simulink model "FBL_UAV_Final_All"  (R2024b)
settings: Solver=ode45  StartTime=0.0  StopTime=3  MaxStep=0.001  RelTol=1e-3
undefined symbols (not defined in the file): A, A_inv, B, Q, R
libraries: slpidlib x8, mpclib x1, rllib x1, simulink x1
(part 1 of 2)
settings Model: Creator=shree  LastModifiedBy=shree
settings SolverCC: MaxConsecutiveMinStep=5
settings RTWCC: GenerateReport=on  LaunchReport=on

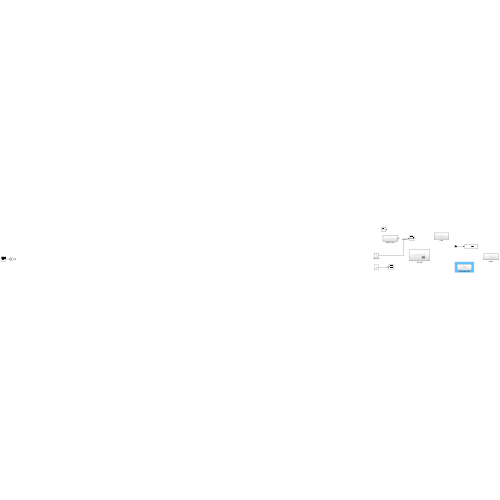
[thumbnail: Simulink's stored preview of the top-level diagram]
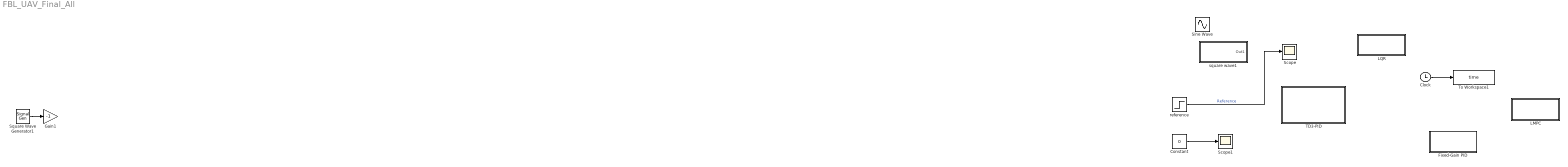
== system FBL_UAV_Final_All ==
  Clock : Clock
      settings: Decimation=4
  Constant : Constant  Value=0
  Fixed-Gain PID : Subsystem
  Gain1 : Gain  Gain=-1
  LMPC : Subsystem
  LQR : Subsystem
  Scope : Scope
  Scope1 : Scope
  Sine Wave : Sin  Amplitude=3  Frequency=3  SampleTime=0
  Square Wave Generator1 : SignalGenerator  WaveForm=square  Amplitude=3
  TD3-PID : Subsystem
  To Workspace1 : ToWorkspace  VariableName=time  SaveFormat=Timeseries  SampleTime=-1
  reference : Step  Time=0.5  SampleTime=0.1
  square wave1 : Subsystem
  wires:
  Square Wave Generator1/1 -> Gain1/1
  Clock/1 -> To Workspace1/1
  Constant/1 -> Scope1/1
  reference/1 -> Scope/1  "Reference"

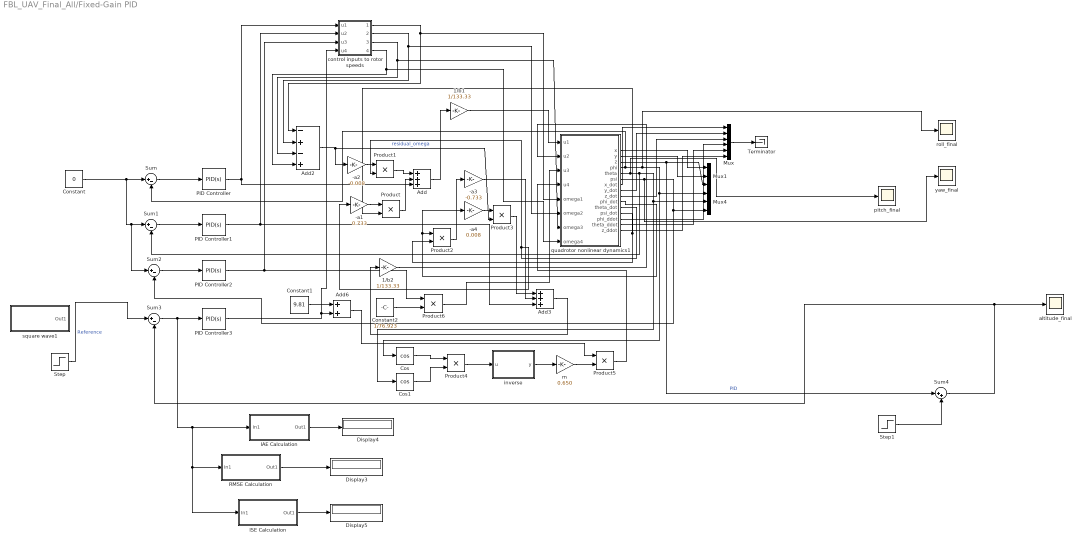
== system FBL_UAV_Final_All/Fixed-Gain PID ==
  -a1 : Gain  Gain=0.733
  -a2 : Gain  Gain=-0.008
  -a3 : Gain  Gain=-0.733
  -a4 : Gain  Gain=0.008
  1/b1 : Gain  Gain=1/133.33
  1/b2 : Gain  Gain=1/133.33
  Add : Sum  Inputs=+++
  Add2 : Sum  Inputs=-+-+
  Add3 : Sum  Inputs=+++
  Add6 : Sum
  Constant : Constant  Value=0
  Constant1 : Constant  Value=9.81
  Constant2 : Constant  Value=1/76.923
  Cos : Trigonometry  Operator=cos
  Cos1 : Trigonometry  Operator=cos
  Display3 : Display
  Display4 : Display
  Display5 : Display
  IAE Calculation : Subsystem
  ISE Calculation : Subsystem
  Mux : Mux  Inputs=6
  Mux1 : Mux  Inputs=3
  Mux4 : Mux  Inputs=3
  PID Controller : slpidlib/PID Controller  Controller=PID  Form=Parallel  TimeDomain=Continuous-time  UseExternalTs=off  SampleTime=-1  IntegratorMethod=Forward Euler  FilterMethod=Forward Euler  ControllerParametersSource=internal  P=50  I=50  UseKiTs=off  D=50  UseExternalDerivativeSource=off  N=200  UseFilter=on  TunerSelectOption=Transfer Function Based (PID Tuner App)  InitialConditionSource=internal  InitialConditionForIntegrator=0  InitialConditionForFilter=0  DifferentiatorICPrevScaledInput=0  ExternalReset=none  TrackingMode=off  Kt=1  LimitOutput=off  SatLimitsSource=internal  UpperSaturationLimit=inf  LowerSaturationLimit=-inf  LinearizeAsGain=on  AntiWindupMode=none  Kb=1  LimitIntegrator=off  UpperIntegratorSaturationLimit=inf  LowerIntegratorSaturationLimit=-inf  POutMin=[]  POutMax=[]  IOutMin=[]  IOutMax=[]  DOutMin=[]  DOutMax=[]  NOutMin=[]  NOutMax=[]  SumOutMin=[]  SumOutMax=[]  SaturationOutMin=[]  SaturationOutMax=[]  PParamMin=[]  PParamMax=[]  IParamMin=[]  IParamMax=[]  DParamMin=[]  DParamMax=[]  NParamMin=[]  NParamMax=[]  KbParamMin=[]  KbParamMax=[]  KtParamMin=[]  KtParamMax=[]  KbOutMin=[]  KbOutMax=[]  KtOutMin=[]  KtOutMax=[]  IntegratorOutMin=[]  IntegratorOutMax=[]  FilterOutMin=[]  FilterOutMax=[]  SumI1OutMin=[]  SumI1OutMax=[]  SumI2OutMin=[]  SumI2OutMax=[]  SumI3OutMin=[]  SumI3OutMax=[]  SumI4OutMin=[]  SumI4OutMax=[]  SumDOutMin=[]  SumDOutMax=[]  DifferentiatorOutMin=[]  DifferentiatorOutMax=[]  FilterDiffOutCoefMin=[]  FilterDiffOutCoefMax=[]  ReciprocalOutMin=[]  ReciprocalOutMax=[]  SumDenOutMin=[]  SumDenOutMax=[]  SumNumOutMin=[]  SumNumOutMax=[]  DivideOutMin=[]  DivideOutMax=[]  UdiffTsProdOutMin=[]  UdiffTsProdOutMax=[]  NTsProdOutMin=[]  NTsProdOutMax=[]  UintegralTsProdOutMin=[]  UintegralTsProdOutMax=[]  UngainTsProdOutMin=[]  UngainTsProdOutMax=[]  ClampingZeroOutDataTypeStr=Inherit: Inherit via back propagation  ClampingZeroOutMin=[]  ClampingZeroOutMax=[]  FilterDenConstantOutDataTypeStr=Inherit: Inherit via back propagation  FilterDenConstantOutMin=[]  FilterDenConstantOutMax=[]  PCopyOutDataTypeStr=Inherit: Inherit via back propagation  PCopyOutMin=[]  PCopyOutMax=[]  NCopyOutDataTypeStr=Inherit: Inherit via back propagation  NCopyOutMin=[]  NCopyOutMax=[]  IntegratorContinuousStateAttributes=''  IntegratorStateMustResolveToSignalObject=off  IntegratorRTWStateStorageClass=Auto  FilterContinuousStateAttributes=''  FilterStateMustResolveToSignalObject=off  FilterRTWStateStorageClass=Auto  ParallelPVariant=InternalParameters  IdealPVariant=Disabled  IVariant=InternalParameters  DVariant=InternalParameters  IntegratorVariant=Continuous  SatVariant=Disabled  AWVariant=Passthrough  PCopyVariant=Disabled  TRVariant=Disabled  FdbkBlocksVariant=Forward  IdealPFdbkVariant=Disabled  SatFdbkVariant=Disabled  DerivativeFilterVariant=ContFilter  NVariant=InternalParameters  NCopyVariant=Disabled  FilterICVariant=InternalICsFilter  IntegratorICVariant=InternalICs  ExternalResetVariant=Disabled  TRSumVariant=Passthrough  SumFdbkVariant=Disabled  SumVariant=Sum_PID  TsampFilterVariant=InternalTs  TsampNgainVariant=Passthrough  TsampIntegralVariant=Disabled_SignalSpec  ExternalSaturationOutDataTypeStr=Inherit: Same as second input  DerivativeSourceVariant=ErrorSignal  PreIntVariant=InternalPreInt
  PID Controller1 : slpidlib/PID Controller  Controller=PID  Form=Parallel  TimeDomain=Continuous-time  UseExternalTs=off  SampleTime=-1  IntegratorMethod=Forward Euler  FilterMethod=Forward Euler  ControllerParametersSource=internal  P=10  I=0.5  UseKiTs=off  D=10  UseExternalDerivativeSource=off  N=100  UseFilter=on  TunerSelectOption=Transfer Function Based (PID Tuner App)  InitialConditionSource=internal  InitialConditionForIntegrator=0  InitialConditionForFilter=0  DifferentiatorICPrevScaledInput=0  ExternalReset=none  TrackingMode=off  Kt=1  LimitOutput=off  SatLimitsSource=internal  UpperSaturationLimit=inf  LowerSaturationLimit=-inf  LinearizeAsGain=on  AntiWindupMode=none  Kb=1  LimitIntegrator=off  UpperIntegratorSaturationLimit=inf  LowerIntegratorSaturationLimit=-inf  POutMin=[]  POutMax=[]  IOutMin=[]  IOutMax=[]  DOutMin=[]  DOutMax=[]  NOutMin=[]  NOutMax=[]  SumOutMin=[]  SumOutMax=[]  SaturationOutMin=[]  SaturationOutMax=[]  PParamMin=[]  PParamMax=[]  IParamMin=[]  IParamMax=[]  DParamMin=[]  DParamMax=[]  NParamMin=[]  NParamMax=[]  KbParamMin=[]  KbParamMax=[]  KtParamMin=[]  KtParamMax=[]  KbOutMin=[]  KbOutMax=[]  KtOutMin=[]  KtOutMax=[]  IntegratorOutMin=[]  IntegratorOutMax=[]  FilterOutMin=[]  FilterOutMax=[]  SumI1OutMin=[]  SumI1OutMax=[]  SumI2OutMin=[]  SumI2OutMax=[]  SumI3OutMin=[]  SumI3OutMax=[]  SumI4OutMin=[]  SumI4OutMax=[]  SumDOutMin=[]  SumDOutMax=[]  DifferentiatorOutMin=[]  DifferentiatorOutMax=[]  FilterDiffOutCoefMin=[]  FilterDiffOutCoefMax=[]  ReciprocalOutMin=[]  ReciprocalOutMax=[]  SumDenOutMin=[]  SumDenOutMax=[]  SumNumOutMin=[]  SumNumOutMax=[]  DivideOutMin=[]  DivideOutMax=[]  UdiffTsProdOutMin=[]  UdiffTsProdOutMax=[]  NTsProdOutMin=[]  NTsProdOutMax=[]  UintegralTsProdOutMin=[]  UintegralTsProdOutMax=[]  UngainTsProdOutMin=[]  UngainTsProdOutMax=[]  ClampingZeroOutDataTypeStr=Inherit: Inherit via back propagation  ClampingZeroOutMin=[]  ClampingZeroOutMax=[]  FilterDenConstantOutDataTypeStr=Inherit: Inherit via back propagation  FilterDenConstantOutMin=[]  FilterDenConstantOutMax=[]  PCopyOutDataTypeStr=Inherit: Inherit via back propagation  PCopyOutMin=[]  PCopyOutMax=[]  NCopyOutDataTypeStr=Inherit: Inherit via back propagation  NCopyOutMin=[]  NCopyOutMax=[]  IntegratorContinuousStateAttributes=''  IntegratorStateMustResolveToSignalObject=off  IntegratorRTWStateStorageClass=Auto  FilterContinuousStateAttributes=''  FilterStateMustResolveToSignalObject=off  FilterRTWStateStorageClass=Auto  ParallelPVariant=InternalParameters  IdealPVariant=Disabled  IVariant=InternalParameters  DVariant=InternalParameters  IntegratorVariant=Continuous  SatVariant=Disabled  AWVariant=Passthrough  PCopyVariant=Disabled  TRVariant=Disabled  FdbkBlocksVariant=Forward  IdealPFdbkVariant=Disabled  SatFdbkVariant=Disabled  DerivativeFilterVariant=ContFilter  NVariant=InternalParameters  NCopyVariant=Disabled  FilterICVariant=InternalICsFilter  IntegratorICVariant=InternalICs  ExternalResetVariant=Disabled  TRSumVariant=Passthrough  SumFdbkVariant=Disabled  SumVariant=Sum_PID  TsampFilterVariant=InternalTs  TsampNgainVariant=Passthrough  TsampIntegralVariant=Disabled_SignalSpec  ExternalSaturationOutDataTypeStr=Inherit: Same as second input  DerivativeSourceVariant=ErrorSignal  PreIntVariant=InternalPreInt
  PID Controller2 : slpidlib/PID Controller  Controller=PID  Form=Parallel  TimeDomain=Continuous-time  UseExternalTs=off  SampleTime=-1  IntegratorMethod=Forward Euler  FilterMethod=Forward Euler  ControllerParametersSource=internal  P=43.  I=4  UseKiTs=off  D=130  UseExternalDerivativeSource=off  N=9  UseFilter=on  TunerSelectOption=Transfer Function Based (PID Tuner App)  InitialConditionSource=internal  InitialConditionForIntegrator=0  InitialConditionForFilter=0  DifferentiatorICPrevScaledInput=0  ExternalReset=none  TrackingMode=off  Kt=1  LimitOutput=off  SatLimitsSource=internal  UpperSaturationLimit=inf  LowerSaturationLimit=-inf  LinearizeAsGain=on  AntiWindupMode=none  Kb=1  LimitIntegrator=off  UpperIntegratorSaturationLimit=inf  LowerIntegratorSaturationLimit=-inf  POutMin=[]  POutMax=[]  IOutMin=[]  IOutMax=[]  DOutMin=[]  DOutMax=[]  NOutMin=[]  NOutMax=[]  SumOutMin=[]  SumOutMax=[]  SaturationOutMin=[]  SaturationOutMax=[]  PParamMin=[]  PParamMax=[]  IParamMin=[]  IParamMax=[]  DParamMin=[]  DParamMax=[]  NParamMin=[]  NParamMax=[]  KbParamMin=[]  KbParamMax=[]  KtParamMin=[]  KtParamMax=[]  KbOutMin=[]  KbOutMax=[]  KtOutMin=[]  KtOutMax=[]  IntegratorOutMin=[]  IntegratorOutMax=[]  FilterOutMin=[]  FilterOutMax=[]  SumI1OutMin=[]  SumI1OutMax=[]  SumI2OutMin=[]  SumI2OutMax=[]  SumI3OutMin=[]  SumI3OutMax=[]  SumI4OutMin=[]  SumI4OutMax=[]  SumDOutMin=[]  SumDOutMax=[]  DifferentiatorOutMin=[]  DifferentiatorOutMax=[]  FilterDiffOutCoefMin=[]  FilterDiffOutCoefMax=[]  ReciprocalOutMin=[]  ReciprocalOutMax=[]  SumDenOutMin=[]  SumDenOutMax=[]  SumNumOutMin=[]  SumNumOutMax=[]  DivideOutMin=[]  DivideOutMax=[]  UdiffTsProdOutMin=[]  UdiffTsProdOutMax=[]  NTsProdOutMin=[]  NTsProdOutMax=[]  UintegralTsProdOutMin=[]  UintegralTsProdOutMax=[]  UngainTsProdOutMin=[]  UngainTsProdOutMax=[]  ClampingZeroOutDataTypeStr=Inherit: Inherit via back propagation  ClampingZeroOutMin=[]  ClampingZeroOutMax=[]  FilterDenConstantOutDataTypeStr=Inherit: Inherit via back propagation  FilterDenConstantOutMin=[]  FilterDenConstantOutMax=[]  PCopyOutDataTypeStr=Inherit: Inherit via back propagation  PCopyOutMin=[]  PCopyOutMax=[]  NCopyOutDataTypeStr=Inherit: Inherit via back propagation  NCopyOutMin=[]  NCopyOutMax=[]  IntegratorContinuousStateAttributes=''  IntegratorStateMustResolveToSignalObject=off  IntegratorRTWStateStorageClass=Auto  FilterContinuousStateAttributes=''  FilterStateMustResolveToSignalObject=off  FilterRTWStateStorageClass=Auto  ParallelPVariant=InternalParameters  IdealPVariant=Disabled  IVariant=InternalParameters  DVariant=InternalParameters  IntegratorVariant=Continuous  SatVariant=Disabled  AWVariant=Passthrough  PCopyVariant=Disabled  TRVariant=Disabled  FdbkBlocksVariant=Forward  IdealPFdbkVariant=Disabled  SatFdbkVariant=Disabled  DerivativeFilterVariant=ContFilter  NVariant=InternalParameters  NCopyVariant=Disabled  FilterICVariant=InternalICsFilter  IntegratorICVariant=InternalICs  ExternalResetVariant=Disabled  TRSumVariant=Passthrough  SumFdbkVariant=Disabled  SumVariant=Sum_PID  TsampFilterVariant=InternalTs  TsampNgainVariant=Passthrough  TsampIntegralVariant=Disabled_SignalSpec  ExternalSaturationOutDataTypeStr=Inherit: Same as second input  DerivativeSourceVariant=ErrorSignal  PreIntVariant=InternalPreInt
  PID Controller3 : slpidlib/PID Controller  Controller=PID  Form=Parallel  TimeDomain=Continuous-time  UseExternalTs=off  SampleTime=-1  IntegratorMethod=Forward Euler  FilterMethod=Forward Euler  ControllerParametersSource=internal  P=100  I=10  UseKiTs=off  D=100  UseExternalDerivativeSource=off  N=100  UseFilter=on  TunerSelectOption=Transfer Function Based (PID Tuner App)  InitialConditionSource=internal  InitialConditionForIntegrator=0  InitialConditionForFilter=0  DifferentiatorICPrevScaledInput=0  ExternalReset=none  TrackingMode=off  Kt=1  LimitOutput=off  SatLimitsSource=internal  UpperSaturationLimit=inf  LowerSaturationLimit=-inf  LinearizeAsGain=on  AntiWindupMode=none  Kb=1  LimitIntegrator=off  UpperIntegratorSaturationLimit=inf  LowerIntegratorSaturationLimit=-inf  POutMin=[]  POutMax=[]  IOutMin=[]  IOutMax=[]  DOutMin=[]  DOutMax=[]  NOutMin=[]  NOutMax=[]  SumOutMin=[]  SumOutMax=[]  SaturationOutMin=[]  SaturationOutMax=[]  PParamMin=[]  PParamMax=[]  IParamMin=[]  IParamMax=[]  DParamMin=[]  DParamMax=[]  NParamMin=[]  NParamMax=[]  KbParamMin=[]  KbParamMax=[]  KtParamMin=[]  KtParamMax=[]  KbOutMin=[]  KbOutMax=[]  KtOutMin=[]  KtOutMax=[]  IntegratorOutMin=[]  IntegratorOutMax=[]  FilterOutMin=[]  FilterOutMax=[]  SumI1OutMin=[]  SumI1OutMax=[]  SumI2OutMin=[]  SumI2OutMax=[]  SumI3OutMin=[]  SumI3OutMax=[]  SumI4OutMin=[]  SumI4OutMax=[]  SumDOutMin=[]  SumDOutMax=[]  DifferentiatorOutMin=[]  DifferentiatorOutMax=[]  FilterDiffOutCoefMin=[]  FilterDiffOutCoefMax=[]  ReciprocalOutMin=[]  ReciprocalOutMax=[]  SumDenOutMin=[]  SumDenOutMax=[]  SumNumOutMin=[]  SumNumOutMax=[]  DivideOutMin=[]  DivideOutMax=[]  UdiffTsProdOutMin=[]  UdiffTsProdOutMax=[]  NTsProdOutMin=[]  NTsProdOutMax=[]  UintegralTsProdOutMin=[]  UintegralTsProdOutMax=[]  UngainTsProdOutMin=[]  UngainTsProdOutMax=[]  ClampingZeroOutDataTypeStr=Inherit: Inherit via back propagation  ClampingZeroOutMin=[]  ClampingZeroOutMax=[]  FilterDenConstantOutDataTypeStr=Inherit: Inherit via back propagation  FilterDenConstantOutMin=[]  FilterDenConstantOutMax=[]  PCopyOutDataTypeStr=Inherit: Inherit via back propagation  PCopyOutMin=[]  PCopyOutMax=[]  NCopyOutDataTypeStr=Inherit: Inherit via back propagation  NCopyOutMin=[]  NCopyOutMax=[]  IntegratorContinuousStateAttributes=''  IntegratorStateMustResolveToSignalObject=off  IntegratorRTWStateStorageClass=Auto  FilterContinuousStateAttributes=''  FilterStateMustResolveToSignalObject=off  FilterRTWStateStorageClass=Auto  ParallelPVariant=InternalParameters  IdealPVariant=Disabled  IVariant=InternalParameters  DVariant=InternalParameters  IntegratorVariant=Continuous  SatVariant=Disabled  AWVariant=Passthrough  PCopyVariant=Disabled  TRVariant=Disabled  FdbkBlocksVariant=Forward  IdealPFdbkVariant=Disabled  SatFdbkVariant=Disabled  DerivativeFilterVariant=ContFilter  NVariant=InternalParameters  NCopyVariant=Disabled  FilterICVariant=InternalICsFilter  IntegratorICVariant=InternalICs  ExternalResetVariant=Disabled  TRSumVariant=Passthrough  SumFdbkVariant=Disabled  SumVariant=Sum_PID  TsampFilterVariant=InternalTs  TsampNgainVariant=Passthrough  TsampIntegralVariant=Disabled_SignalSpec  ExternalSaturationOutDataTypeStr=Inherit: Same as second input  DerivativeSourceVariant=ErrorSignal  PreIntVariant=InternalPreInt
  Product{,1..6} (7 alike) : Product
  RMSE Calculation : Subsystem
  Step : Step  Time=0.5  SampleTime=0
  Step1 : Step  After=0.1  SampleTime=0
  Sum{,1..3} (4 alike) : Sum  Inputs=|+-
  Sum4 : Sum  Inputs=|++
  Terminator : Terminator
  altitude_final : Scope
  control inputs to rotor speeds : Subsystem
  inverse : MATLAB Function  TreatAsAtomicUnit=on
  m : Gain  Gain=0.650
  pitch_final : Scope
  quadrotor nonlinear dynamics1 : Subsystem
  roll_final : Scope
  square wave1 : Subsystem
  yaw_final : Scope
  wires:
  quadrotor nonlinear dynamics1/15(z_ddot) -> Mux/6
  quadrotor nonlinear dynamics1/13(phi_ddot) -> Mux/4
  control inputs to rotor speeds/2(omega2) -> quadrotor nonlinear dynamics1/6(omega2), Add2/2
  Product2/1 -> -a3/1
  -a4/1 -> Product3/1
  Product4/1 -> inverse/1(u)
  Add3/1 -> 1/b2/1
  Step/1 -> Sum3/1  "Reference"
  quadrotor nonlinear dynamics1/1(x) -> Mux1/1
  Product3/1 -> Add3/1
  PID Controller2/1 -> control inputs to rotor speeds/3(u3), Product6/1
  quadrotor nonlinear dynamics1/11(theta_dot) -> Product1/2, -a1/1
  Add2/1 -> -a2/1, Product3/2  "residual_omega"
  Sum3/1 -> ISE Calculation/1(In1), RMSE Calculation/1(In1), IAE Calculation/1(In1), PID Controller3/1
  Constant/1 -> Sum2/1, Sum1/1, Sum/1
  IAE Calculation/1(Out1) -> Display4/1
  Add6/1 -> Product5/1
  inverse/1(y) -> m/1
  1/b2/1 -> quadrotor nonlinear dynamics1/2(u2)
  control inputs to rotor speeds/3(omega3) -> quadrotor nonlinear dynamics1/7(omega3), Add2/3
  control inputs to rotor speeds/1(omega1) -> quadrotor nonlinear dynamics1/5(omega1), Add2/1
  Sum/1 -> PID Controller/1
  -a3/1 -> Add3/2
  Product1/1 -> Add/1
  PID Controller3/1 -> control inputs to rotor speeds/4(u4), Add6/2
  quadrotor nonlinear dynamics1/12(psi_dot) -> Product2/2, Product/2
  quadrotor nonlinear dynamics1/5(theta) -> pitch_final/1, Sum1/2, Mux4/2, Cos1/1
  -a1/1 -> Product/1
  Product6/1 -> quadrotor nonlinear dynamics1/3(u3)
  PID Controller/1 -> Add/3, control inputs to rotor speeds/1(u1)
  quadrotor nonlinear dynamics1/8(y_dot) -> Mux/2
  quadrotor nonlinear dynamics1/9(z_dot) -> Mux/3
  quadrotor nonlinear dynamics1/14(theta_ddot) -> Mux/5
  quadrotor nonlinear dynamics1/2(y) -> Mux1/2
  control inputs to rotor speeds/4(omega4) -> quadrotor nonlinear dynamics1/8(omega4), Add2/4
  Product/1 -> Add/2
  quadrotor nonlinear dynamics1/6(psi) -> yaw_final/1, Sum2/2, Mux4/3
  ISE Calculation/1(Out1) -> Display5/1
  Product5/1 -> quadrotor nonlinear dynamics1/4(u4)
  Constant2/1 -> Product6/2
  Sum2/1 -> PID Controller2/1
  quadrotor nonlinear dynamics1/3(z) -> Sum4/1, Mux1/3  "PID"
  1/b1/1 -> quadrotor nonlinear dynamics1/1(u1)
  Mux/1 -> Terminator/1
  Constant1/1 -> Add6/1
  Sum1/1 -> PID Controller1/1
  Cos1/1 -> Product4/2
  -a2/1 -> Product1/1
  Add/1 -> 1/b1/1
  quadrotor nonlinear dynamics1/7(x_dot) -> Mux/1
  quadrotor nonlinear dynamics1/4(phi) -> Sum/2, roll_final/1, Cos/1, Mux4/1
  PID Controller1/1 -> control inputs to rotor speeds/2(u2), Add3/3
  RMSE Calculation/1(Out1) -> Display3/1
  quadrotor nonlinear dynamics1/10(phi_dot) -> -a4/1, Product2/1
  m/1 -> Product5/2
  Cos/1 -> Product4/1
  Step1/1 -> Sum4/2
  Sum4/1 -> altitude_final/1, Sum3/2

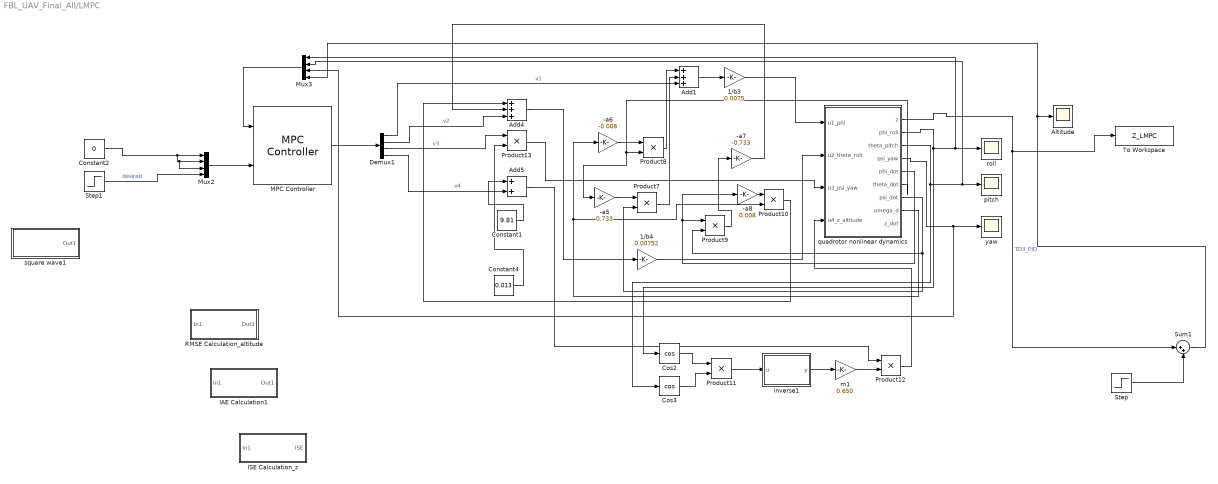
== system FBL_UAV_Final_All/LMPC ==
  -a5 : Gain  Gain=0.733
  -a6 : Gain  Gain=-0.008
  -a7 : Gain  Gain=-0.733
  -a8 : Gain  Gain=0.008
  1/b3 : Gain  Gain=0.0075
  1/b4 : Gain  Gain=0.00752
  Add1 : Sum  Inputs=+++
  Add4 : Sum  Inputs=+++
  Add5 : Sum
  Altitude : Scope
  Constant1 : Constant  Value=9.81
  Constant2 : Constant  Value=0
  Constant4 : Constant  Value=0.013
  Cos2 : Trigonometry  Operator=cos
  Cos3 : Trigonometry  Operator=cos
  Demux1 : Demux
  IAE Calculation1 : Subsystem
  ISE Calculation_z : Subsystem
  MPC Controller : mpclib/MPC Controller  SCDEnableBlockLinearizationSpecification=on  mpcobj=mpc1  is_multiple=0  enable_value=0  return_u0=off  updateMPCinCallerWorkspace=on  md_inport=off  mv_inport=off  uref_inport=off  return_cost=off  return_mvseq=off  return_qpstatus=off  return_xseq=off  return_state=off  return_ovseq=off  state_inport=off  umin_inport=off  umax_inport=off  ymin_inport=off  ymax_inport=off  cc_inport=off  ywt_inport=off  uwt_inport=off  duwt_inport=off  rhoeps_inport=off  pm_inport=off  MaximumP=10  HorizonChoice=FixedHorizon  n_ts=0.01  n_p=10  n_mv=4  n_md=0  n_ud=0  n_mo=4  n_uo=0  BlockDataType=double  SampleTimeInherited=off  switch_inport=off
  Mux2 : Mux
  Mux3 : Mux
  Product{7..13} (7 alike) : Product
  RMSE Calculation_altitude : Subsystem
  Step : Step  After=0.1  SampleTime=0
  Step1 : Step  Time=0.5  SampleTime=0
  Sum1 : Sum  Inputs=|++
  To Workspace : ToWorkspace  VariableName=Z_LMPC  SaveFormat=Timeseries  SampleTime=-1
  inverse1 : MATLAB Function  TreatAsAtomicUnit=on
  m1 : Gain  Gain=0.650
  pitch : Scope
  quadrotor nonlinear dynamics : Subsystem
  roll : Scope
  square wave1 : Subsystem
  yaw : Scope
  wires:
  1/b3/1 -> quadrotor nonlinear dynamics/1(u1_phi)
  -a6/1 -> Product8/1
  quadrotor nonlinear dynamics/2(phi_roll) -> Cos2/1, Mux3/1, roll/1
  MPC Controller/1 -> Demux1/1
  Product7/1 -> Add1/2
  Product10/1 -> Add4/1
  quadrotor nonlinear dynamics/6(theta_dot) -> -a5/1, Product8/2
  Constant1/1 -> Add5/1
  Cos3/1 -> Product11/2
  Product13/1 -> quadrotor nonlinear dynamics/3(u3_psi_yaw)
  Product11/1 -> inverse1/1(u)
  Product12/1 -> quadrotor nonlinear dynamics/4(u4_z_altitude)
  Cos2/1 -> Product11/1
  Demux1/1 -> Add1/3  "v1"
  Product9/1 -> -a7/1
  -a8/1 -> Product10/1
  quadrotor nonlinear dynamics/3(theta_pitch) -> Mux3/2, pitch/1, Cos3/1
  quadrotor nonlinear dynamics/4(psi_yaw) -> Mux3/3, yaw/1
  Add4/1 -> 1/b4/1
  1/b4/1 -> quadrotor nonlinear dynamics/2(u2_theta_roll)
  Demux1/3 -> Product13/1  "v3"
  Constant4/1 -> Product13/2
  Mux3/1 -> MPC Controller/1
  quadrotor nonlinear dynamics/5(phi_dot) -> -a8/1, Product9/1
  m1/1 -> Product12/2
  Add5/1 -> Product12/1
  Demux1/2 -> Add4/3  "v2"
  quadrotor nonlinear dynamics/8(omega_d) -> Product10/2, -a6/1
  inverse1/1(y) -> m1/1
  Product8/1 -> Add1/1
  Constant2/1 -> Mux2/3, Mux2/2, Mux2/1
  -a5/1 -> Product7/1
  quadrotor nonlinear dynamics/7(psi_dot) -> Product9/2, Product7/2
  Mux2/1 -> MPC Controller/2
  Add1/1 -> 1/b3/1
  Demux1/4 -> Add5/2  "v4"
  Step1/1 -> Mux2/4  "desired"
  -a7/1 -> Add4/2
  quadrotor nonlinear dynamics/1(z) -> Sum1/1, To Workspace/1  "TD3_PID"
  Step/1 -> Sum1/2
  Sum1/1 -> Mux3/4, Altitude/1

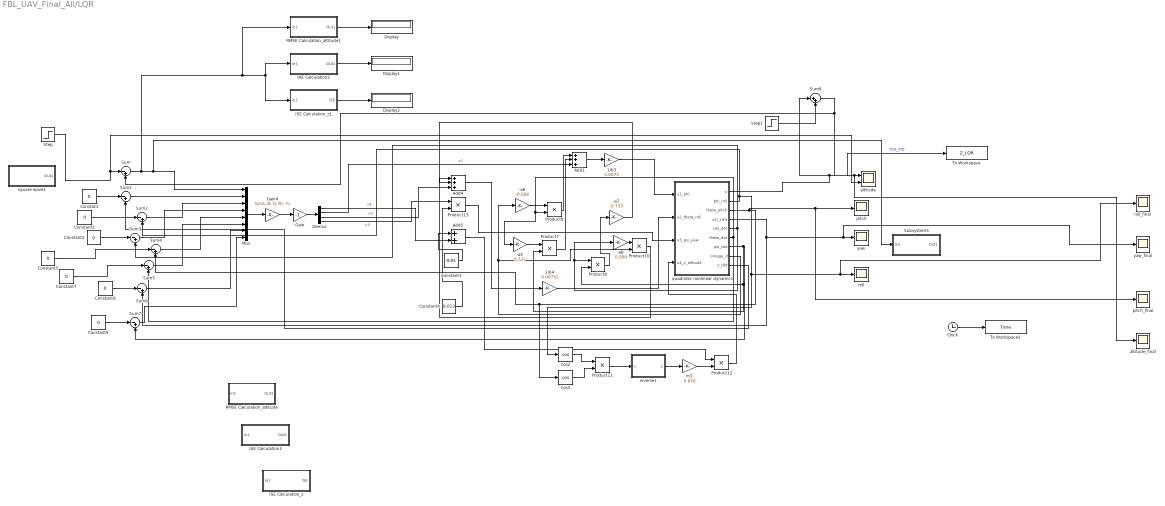
== system FBL_UAV_Final_All/LQR ==
  -a5 : Gain  Gain=0.733
  -a6 : Gain  Gain=-0.008
  -a7 : Gain  Gain=-0.733
  -a8 : Gain  Gain=0.008
  1/b3 : Gain  Gain=0.0075
  1/b4 : Gain  Gain=0.00752
  Add1 : Sum  Inputs=+++
  Add4 : Sum  Inputs=+++
  Add5 : Sum
  Clock : Clock
  Constant{,1..2,5,7..9} (7 alike) : Constant  Value=0
  Constant3 : Constant  Value=9.81
  Constant4 : Constant  Value=0.013
  Cos2 : Trigonometry  Operator=cos
  Cos3 : Trigonometry  Operator=cos
  Demux : Demux
  Display : Display
  Display1 : Display
  Display2 : Display
  Gain : Gain  Gain=-1
  Gain4 : Gain  Gain=lqr(A, B, Q, R);  Multiplication=Matrix(K*u)
  IAE Calculation1 : Subsystem
  IAE Calculation2 : Subsystem
  ISE Calculation_z : Subsystem
  ISE Calculation_z1 : Subsystem
  Mux : Mux  Inputs=8
  Product{7..13} (7 alike) : Product
  RMSE Calculation_altitude : Subsystem
  RMSE Calculation_altitude1 : Subsystem
  Step : Step  Time=0.5  SampleTime=0
  Step1 : Step  After=0.1  SampleTime=0
  Subsystem5 : Subsystem
  Sum{,1..7} (8 alike) : Sum  Inputs=|-+
  Sum8 : Sum  Inputs=|++
  To Workspace : ToWorkspace  VariableName=Z_LQR  SaveFormat=Timeseries  SampleTime=-1
  To Workspace2 : ToWorkspace  VariableName=Time  SaveFormat=Timeseries  SampleTime=-1
  altitude : Scope  NumInputPorts=2
  altitude_final : Scope
  inverse1 : MATLAB Function  TreatAsAtomicUnit=on
  m1 : Gain  Gain=0.650
  pitch : Scope
  pitch_final : Scope
  quadrotor nonlinear dynamics : Subsystem
  roll : Scope
  roll_final : Scope
  square wave1 : Subsystem
  yaw : Scope
  yaw_final : Scope
  wires:
  Demux/2 -> Add1/3  "v1"
  Demux/3 -> Add4/3  "v2"
  Constant5/1 -> Sum4/1
  Add1/1 -> 1/b3/1
  Add4/1 -> 1/b4/1
  Product9/1 -> -a7/1
  quadrotor nonlinear dynamics/2(phi_roll) -> Sum2/2, roll_final/1, roll/1, Cos2/1
  inverse1/1(y) -> m1/1
  quadrotor nonlinear dynamics/8(omega_d) -> Product10/2, -a6/1
  quadrotor nonlinear dynamics/6(theta_dot) -> Sum5/2, -a5/1, Product8/2
  Add5/1 -> Product12/1
  quadrotor nonlinear dynamics/3(theta_pitch) -> Sum4/2, Cos3/1, pitch_final/1, pitch/1
  -a5/1 -> Product7/1
  Cos2/1 -> Product11/1
  -a7/1 -> Add4/2
  Product8/1 -> Add1/1
  Product7/1 -> Add1/2
  Constant4/1 -> Product13/2
  quadrotor nonlinear dynamics/5(phi_dot) -> Sum3/2, -a8/1, Product9/1
  Product12/1 -> quadrotor nonlinear dynamics/4(u4_z_altitude)
  Constant7/1 -> Sum5/1
  quadrotor nonlinear dynamics/7(psi_dot) -> Sum7/2, Product9/2, Product7/2
  Constant1/1 -> Sum2/1
  quadrotor nonlinear dynamics/9(z_dot) -> Sum1/2
  Sum7/1 -> Mux/8
  Sum1/1 -> Mux/2
  Cos3/1 -> Product11/2
  quadrotor nonlinear dynamics/4(psi_yaw) -> Sum6/2, yaw_final/1, yaw/1
  Mux/1 -> Gain4/1
  Constant3/1 -> Add5/1
  Sum5/1 -> Mux/6
  Sum6/1 -> Mux/7
  Product10/1 -> Add4/1
  Product11/1 -> inverse1/1(u)
  Clock/1 -> To Workspace2/1
  1/b4/1 -> quadrotor nonlinear dynamics/2(u2_theta_roll)
  Sum2/1 -> Mux/3
  Constant8/1 -> Sum6/1
  Step/1 -> altitude/2, Sum/1
  -a6/1 -> Product8/1
  -a8/1 -> Product10/1
  Constant2/1 -> Sum3/1
  quadrotor nonlinear dynamics/1(z) -> Sum8/1, To Workspace/1  "TD3_PID"
  m1/1 -> Product12/2
  Constant/1 -> Sum1/1
  Sum3/1 -> Mux/4
  Demux/1 -> Add5/2  "v4"
  1/b3/1 -> quadrotor nonlinear dynamics/1(u1_phi)
  Sum4/1 -> Mux/5
  Gain4/1 -> Gain/1
  Constant9/1 -> Sum7/1
  Product13/1 -> quadrotor nonlinear dynamics/3(u3_psi_yaw)
  Demux/4 -> Product13/1  "v3"
  RMSE Calculation_altitude1/1(Out1) -> Display/1
  IAE Calculation2/1(Out1) -> Display1/1
  ISE Calculation_z1/1(ISE) -> Display2/1
  Sum/1 -> RMSE Calculation_altitude1/1(In1), ISE Calculation_z1/1(In1), IAE Calculation2/1(In1), Subsystem5/1(In1), Mux/1
  Gain/1 -> Demux/1
  Step1/1 -> Sum8/2
  Sum8/1 -> altitude_final/1, altitude/1, Sum/2

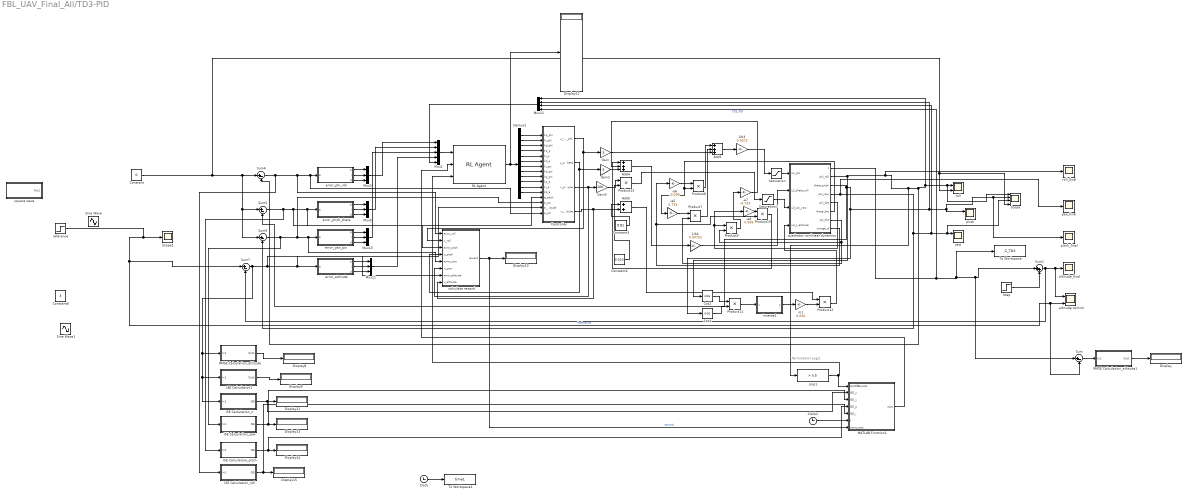
== system FBL_UAV_Final_All/TD3-PID ==
  note: Termination Logic
  -a5 : Gain  Gain=0.733
  -a6 : Gain  Gain=-0.008
  -a7 : Gain  Gain=-0.733
  -a8 : Gain  Gain=0.008
  1/b3 : Gain  Gain=0.0075
  1/b4 : Gain  Gain=0.00752
  Add1 : Sum  Inputs=+++
  Add4 : Sum  Inputs=+++
  Add5 : Sum
  Clock : Clock
      settings: Decimation=4
  Clock2 : Clock
  Constant : Constant  Value=0
  Constant3 : Constant  Value=9.81
  Constant4 : Constant  Value=0.013
  Constant6 : Constant  Value=3
  Controller : Subsystem
  Cos2 : Trigonometry  Operator=cos
  Cos3 : Trigonometry  Operator=cos
  Demux1 : Demux  Outputs=12
  Display{,8..15} (9 alike) : Display
  Gain : Gain  Gain=3
  Gain2 : Gain  Gain=5
  Gain3 : Gain  Gain=100
  IAE Calculation1 : Subsystem
  ISE Calculation_pitch : Subsystem
  ISE Calculation_roll : Subsystem
  ISE Calculation_yaw : Subsystem
  ISE Calculation_z : Subsystem
  MATLAB Function1 : MATLAB Function  TreatAsAtomicUnit=on  SystemSampleTime=0.1
  Mux{3,9..11} (4 alike) : Mux  Inputs=3
  Mux12 : Mux
  Mux2 : Mux  Inputs=5
  Product{7..13} (7 alike) : Product
  RL Agent : rllib/RL Agent  Agent=agent_TD3_Final  ExternalActionAsInput=off  ProvideLastAction=off  ProvideCumRwd=off  TreatAsDirectFeedthrough=on  UseStrictObservationDataTypes=off
  RMSE Calculation_altitude : Subsystem
  RMSE Calculation_altitude1 : Subsystem
  Saturation : Saturate  UpperLimit=30  LowerLimit=-30
  Saturation1 : Saturate  UpperLimit=30  LowerLimit=-30
  Scope : Scope  NumInputPorts=4
  Scope1 : Scope
  Sine Wave : Sin  Amplitude=3  Frequency=3  SampleTime=0
  Sine Wave1 : Sin  Amplitude=3  SampleTime=0
  Step : Step  After=0.1  SampleTime=0
  Sum{,4..7} (5 alike) : Sum  Inputs=|+-
  Sum1 : Sum  Inputs=|++
  To Workspace : ToWorkspace  VariableName=Z_TD3  SaveFormat=Timeseries  SampleTime=-1
  To Workspace1 : ToWorkspace  VariableName=time1  SaveFormat=Timeseries  SampleTime=-1
  altitude control : Scope  NumInputPorts=2
  altitude_final : Scope
  calculate reward : Subsystem
  cmp1 : simulink/Logic and Bit Operations/Compare To Constant  relop=>  const=3.5  OutDataTypeStr=boolean
  error_altitude : Subsystem
  error_phi_roll : Subsystem
  error_pitch_theta : Subsystem
  error_yaw_psi : Subsystem
  inverse1 : MATLAB Function  TreatAsAtomicUnit=on
  m1 : Gain  Gain=0.650
  pitch : Scope  NumInputPorts=2
  pitch_final : Scope
  quadrotor nonlinear dynamics : Subsystem
  reference : Step  Time=0.5  SampleTime=0.1
  roll : Scope  NumInputPorts=2
  roll_final : Scope
  square wave : Subsystem
  yaw : Scope  NumInputPorts=2
  yaw_final : Scope
  wires:
  Constant/1 -> roll/2, Scope/4, Sum6/1, Sum5/1, Sum4/1
  quadrotor nonlinear dynamics/3(theta_pitch) -> Sum5/2, Mux12/2, pitch_final/1, Scope/2, pitch/1, Cos3/1
  quadrotor nonlinear dynamics/2(phi_roll) -> roll_final/1, cmp1/1, Sum4/2, Mux12/1, Scope/1, roll/1, Cos2/1
  1/b3/1 -> Saturation/1
  Gain2/1 -> Add4/3
  Mux9/1 -> Mux2/2
  quadrotor nonlinear dynamics/1(z) -> Sum1/1, Sum/1, To Workspace/1, Mux12/4  "TD3_PID"
  Product12/1 -> quadrotor nonlinear dynamics/4(u4_z_altitude)
  Demux1/1 -> Controller/1(kp_phi)
  ISE Calculation_roll/1(ISE) -> MATLAB Function1/5(ISE_r), Display15/1
  cmp1/1 -> MATLAB Function1/1(OutOfBounds), RL Agent/3
  Sum5/1 -> ISE Calculation_pitch/1(In1), calculate reward/3(error_pitch), Controller/13(e_pitch), error_pitch_theta/1(e)
  calculate reward/1(reward) -> MATLAB Function1/7(input_cost), Display10/1  "reward"
  Demux1/5 -> Controller/5(ki_p)
  Sum6/1 -> ISE Calculation_yaw/1(In1), Controller/14(e_psi), calculate reward/5(error_yaw), error_yaw_psi/1(e)
  Controller/4(u_altitude) -> Add5/2, calculate reward/8(u_altitude)
  Demux1/3 -> Controller/3(kd_phi)
  quadrotor nonlinear dynamics/4(psi_yaw) -> yaw_final/1, Sum6/2, Scope/3, yaw/1, Mux12/3
  Product11/1 -> inverse1/1(u)
  RL Agent/1 -> Display12/1, Demux1/1
  error_yaw_psi/3(d) -> Mux10/3
  Demux1/2 -> Controller/2(ki_phi)
  error_pitch_theta/2(i) -> Mux9/2
  ISE Calculation_yaw/1(ISE) -> MATLAB Function1/3(ISE_y), Display13/1
  Clock2/1 -> MATLAB Function1/6(t)
  Saturation1/1 -> quadrotor nonlinear dynamics/3(u3_psi_yaw)
  Product7/1 -> Add1/2
  -a6/1 -> Product8/1
  Controller/1(u_roll_phii) -> calculate reward/2(u_roll), Gain/1
  Demux1/12 -> Controller/12(kd_a)
  Gain3/1 -> Product13/1
  Mux11/1 -> Mux2/4
  Controller/3(u_psi_yaw) -> Gain3/1, calculate reward/6(u_yaw)
  Mux3/1 -> Mux2/1
  error_pitch_theta/3(d) -> Mux9/3
  Demux1/6 -> Controller/6(kd_p)
  1/b4/1 -> quadrotor nonlinear dynamics/2(u2_theta_roll)
  -a7/1 -> Add4/2
  quadrotor nonlinear dynamics/5(phi_dot) -> -a8/1, Product9/1
  Controller/2(u_pitch_theta) -> calculate reward/4(u_pitch), Gain2/1
  quadrotor nonlinear dynamics/7(psi_dot) -> Product9/2, Product7/2
  Sum4/1 -> ISE Calculation_roll/1(In1), calculate reward/1(error_roll), Controller/16(e_phi), error_phi_roll/1(e)
  Add5/1 -> Product12/1
  Product9/1 -> -a7/1
  Demux1/7 -> Controller/7(ki_psi)
  error_altitude/3(d) -> Mux11/3
  Product10/1 -> Add4/1
  Cos2/1 -> Product11/1
  Sum7/1 -> ISE Calculation_z/1(In1), IAE Calculation1/1(In1), RMSE Calculation_altitude/1(In1), Controller/15(e_altitude), calculate reward/7(error_altitude), error_altitude/1(e)
  Cos3/1 -> Product11/2
  Product13/1 -> Saturation1/1
  MATLAB Function1/1(cost) -> RL Agent/2
  Add4/1 -> 1/b4/1
  Gain/1 -> Add1/3
  m1/1 -> Product12/2
  Mux12/1 -> Mux2/5
  error_phi_roll/1(p) -> Mux3/1
  IAE Calculation1/1(Out1) -> Display9/1
  Demux1/10 -> Controller/10(kp_a)
  Saturation/1 -> quadrotor nonlinear dynamics/1(u1_phi)
  RMSE Calculation_altitude/1(Out1) -> Display8/1
  quadrotor nonlinear dynamics/8(omega_d) -> Product10/2, -a6/1
  Constant4/1 -> Product13/2
  Demux1/4 -> Controller/4(kp_p)
  error_pitch_theta/1(p) -> Mux9/1
  Demux1/9 -> Controller/9(kp_psi)
  error_altitude/2(i) -> Mux11/2
  Constant3/1 -> Add5/1
  inverse1/1(y) -> m1/1
  Add1/1 -> 1/b3/1
  error_yaw_psi/1(p) -> Mux10/1
  -a8/1 -> Product10/1
  error_phi_roll/2(i) -> Mux3/2
  Mux10/1 -> Mux2/3
  Mux2/1 -> RL Agent/1
  -a5/1 -> Product7/1
  ISE Calculation_z/1(ISE) -> MATLAB Function1/2(ISE_z), Display11/1
  quadrotor nonlinear dynamics/6(theta_dot) -> -a5/1, Product8/2
  Demux1/8 -> Controller/8(kd_psi)
  error_phi_roll/3(d) -> Mux3/3
  error_altitude/1(p) -> Mux11/1
  Demux1/11 -> Controller/11(ki_a)
  ISE Calculation_pitch/1(ISE) -> MATLAB Function1/4(ISE_p), Display14/1
  error_yaw_psi/2(i) -> Mux10/2
  Product8/1 -> Add1/1
  Clock/1 -> To Workspace1/1
  reference/1 -> altitude control/2, Sum/2, Sum7/1, Scope1/1  "Reference"
  Sum/1 -> RMSE Calculation_altitude1/1(In1)
  RMSE Calculation_altitude1/1(Out1) -> Display/1
  Sum1/1 -> altitude control/1, altitude_final/1, Sum7/2
  Step/1 -> Sum1/2

== system FBL_UAV_Final_All/square wave1 ==
  Scope : Scope
  Step : Step  Time=4  SampleTime=0
  Step1 : Step  Time=8  After=-1  SampleTime=0
  Step2 : Step  Time=10  After=-1  SampleTime=0
  Sum6 : Sum  Inputs=|++++
  new : Step  Time=2  SampleTime=0.1
  Out1 : Outport
  wires:
  Sum6/1 -> Out1/1, Scope/1
  Step/1 -> Sum6/2
  new/1 -> Sum6/1
  Step1/1 -> Sum6/3
  Step2/1 -> Sum6/4

== system FBL_UAV_Final_All/Fixed-Gain PID/IAE Calculation ==
  In1 : Inport
  Abs : Abs  SaturateOnIntegerOverflow=off
  Integrator6 : Integrator
  Out1 : Outport
  wires:
  Abs/1 -> Integrator6/1
  Integrator6/1 -> Out1/1
  In1/1 -> Abs/1

== system FBL_UAV_Final_All/Fixed-Gain PID/ISE Calculation ==
  In1 : Inport
  Integrator6 : Integrator
  Square : Math  Operator=square
  Out1 : Outport
  wires:
  Square/1 -> Integrator6/1
  Integrator6/1 -> Out1/1
  In1/1 -> Square/1

== system FBL_UAV_Final_All/Fixed-Gain PID/RMSE Calculation ==
  In1 : Inport
  Gain : Gain  Gain=1/3435
  Memory : Memory
  Sqrt : Sqrt
  Square : Math  Operator=square
  Sum : Sum  Inputs=|++
  Out1 : Outport
  wires:
  In1/1 -> Square/1
  Square/1 -> Sum/1
  Memory/1 -> Sum/2
  Sum/1 -> Gain/1
  Gain/1 -> Sqrt/1, Memory/1
  Sqrt/1 -> Out1/1

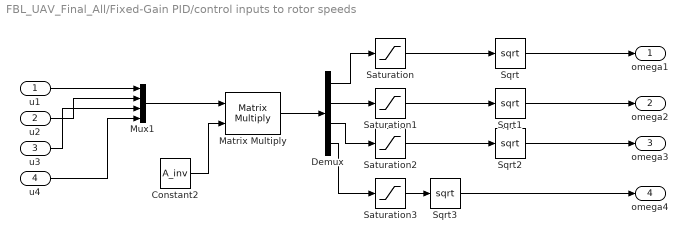
== system FBL_UAV_Final_All/Fixed-Gain PID/control inputs to rotor speeds ==
  u1 : Inport
  u2 : Inport  Port=2
  u3 : Inport  Port=3
  u4 : Inport  Port=4
  Constant2 : Constant  Value=A_inv
  Demux : Demux
  Matrix Multiply : Product  Multiplication=Matrix(*)
  Mux1 : Mux
  Saturation{,1..3} (4 alike) : Saturate  UpperLimit=360000  LowerLimit=0
  Sqrt{,1..3} (4 alike) : Sqrt
  omega1 : Outport
  omega2 : Outport  Port=2
  omega3 : Outport  Port=3
  omega4 : Outport  Port=4
  wires:
  Demux/1 -> Saturation/1
  u1/1 -> Mux1/1
  Demux/2 -> Saturation1/1
  u2/1 -> Mux1/2
  Saturation3/1 -> Sqrt3/1
  Saturation2/1 -> Sqrt2/1
  Saturation/1 -> Sqrt/1
  Matrix Multiply/1 -> Demux/1
  Mux1/1 -> Matrix Multiply/1
  u4/1 -> Mux1/4
  Constant2/1 -> Matrix Multiply/2
  Saturation1/1 -> Sqrt1/1
  Demux/3 -> Saturation2/1
  Demux/4 -> Saturation3/1
  Sqrt2/1 -> omega3/1
  Sqrt/1 -> omega1/1
  u3/1 -> Mux1/3
  Sqrt3/1 -> omega4/1
  Sqrt1/1 -> omega2/1

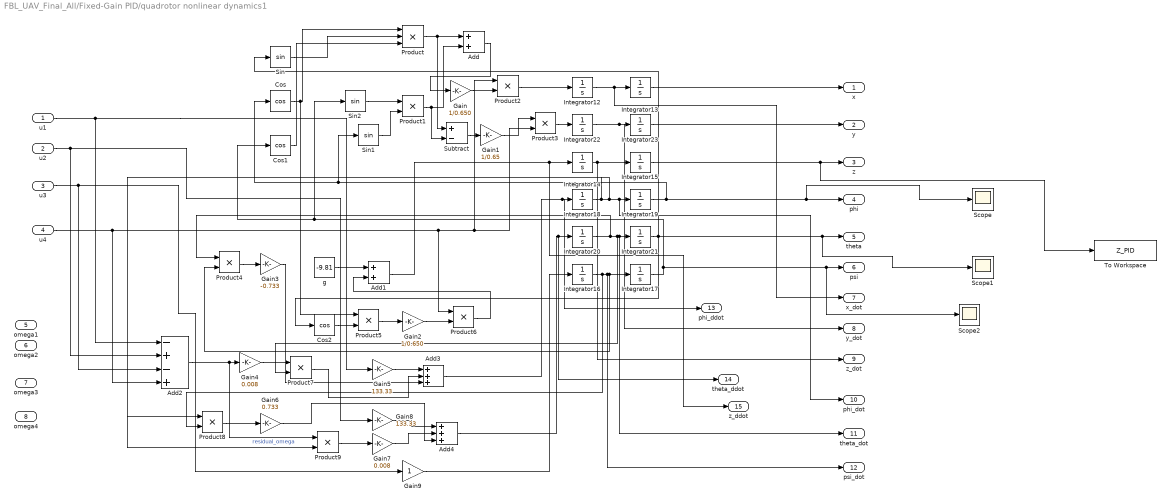
== system FBL_UAV_Final_All/Fixed-Gain PID/quadrotor nonlinear dynamics1 ==
  u1 : Inport
  u2 : Inport  Port=2
  u3 : Inport  Port=3
  u4 : Inport  Port=4
  omega1 : Inport  Port=5
  omega2 : Inport  Port=6
  omega3 : Inport  Port=7
  omega4 : Inport  Port=8
  Add : Sum
  Add1 : Sum
  Add2 : Sum  Inputs=-+-+
  Add3 : Sum  Inputs=+++
  Add4 : Sum  Inputs=+++
  Cos : Trigonometry  Operator=cos
  Cos1 : Trigonometry  Operator=cos
  Cos2 : Trigonometry  Operator=cos
  Gain : Gain  Gain=1/0.650
  Gain1 : Gain  Gain=1/0.65
  Gain2 : Gain  Gain=1/0.650
  Gain3 : Gain  Gain=-0.733
  Gain4 : Gain  Gain=0.008
  Gain5 : Gain  Gain=133.33
  Gain6 : Gain  Gain=0.733
  Gain7 : Gain  Gain=0.008
  Gain8 : Gain  Gain=133.33
  Gain9 : Gain
  Integrator{12..16,18,20,22..23} (9 alike) : Integrator
  Integrator17 : Integrator  InitialCondition=1  LowerSaturationLimit=0
  Integrator19 : Integrator  InitialCondition=1  LowerSaturationLimit=0
  Integrator21 : Integrator  InitialCondition=1  LowerSaturationLimit=0
  Product : Product  Inputs=3
  Product{1..9} (9 alike) : Product
  Scope : Scope
  Scope1 : Scope
  Scope2 : Scope
  Sin : Trigonometry
  Sin1 : Trigonometry
  Sin2 : Trigonometry
  Subtract : Sum  Inputs=+-
  To Workspace : ToWorkspace  VariableName=Z_PID  SaveFormat=Timeseries  SampleTime=-1
  g : Constant  Value=-9.81
  x : Outport
  y : Outport  Port=2
  z : Outport  Port=3
  phi : Outport  Port=4
  theta : Outport  Port=5
  psi : Outport  Port=6
  x_dot : Outport  Port=7
  y_dot : Outport  Port=8
  z_dot : Outport  Port=9
  phi_dot : Outport  Port=10
  theta_dot : Outport  Port=11
  psi_dot : Outport  Port=12
  phi_ddot : Outport  Port=13
  theta_ddot : Outport  Port=14
  z_ddot : Outport  Port=15
  wires:
  Gain9/1 -> Integrator16/1
  Product9/1 -> Gain7/1
  Gain6/1 -> Add4/3
  Add3/1 -> phi_ddot/1, Integrator18/1
  Add4/1 -> theta_ddot/1, Integrator20/1
  Gain7/1 -> Add4/2
  u3/1 -> Add2/3, Gain9/1
  Add2/1 -> Product9/1, Gain4/1  "residual_omega"
  Gain4/1 -> Product7/1
  u2/1 -> Add2/2, Gain8/1
  Product7/1 -> Add3/2
  Product1/1 -> Subtract/2, Add/2
  g/1 -> Add1/1
  Gain1/1 -> Product3/1
  Integrator18/1 -> Product9/2, Product8/1, phi_dot/1, Integrator19/1
  Gain2/1 -> Product6/2
  Gain8/1 -> Add4/1
  Gain/1 -> Product2/2
  Gain5/1 -> Add3/1
  Product5/1 -> Gain2/1
  Integrator12/1 -> x_dot/1, Integrator13/1
  Product/1 -> Subtract/1, Add/1
  Product2/1 -> Integrator12/1
  Integrator19/1 -> Sin1/1, Cos/1, Scope/1, phi/1
  Integrator15/1 -> To Workspace/1, z/1
  Integrator22/1 -> y_dot/1, Integrator23/1
  Add1/1 -> z_ddot/1, Integrator14/1
  Integrator14/1 -> Integrator15/1, z_dot/1
  Cos1/1 -> Product/3
  Cos/1 -> Product5/1, Product/1
  Integrator23/1 -> y/1
  Integrator17/1 -> Sin2/1, Cos1/1, Scope2/1, psi/1
  Sin1/1 -> Product1/2
  Integrator20/1 -> theta_dot/1, Integrator21/1, Product7/2, Product4/1
  Integrator16/1 -> Product8/2, Integrator17/1, Product4/2, psi_dot/1
  u4/1 -> Add2/4, Product6/1, Product3/2, Product2/1
  Integrator21/1 -> Scope1/1, theta/1, Cos2/1, Sin/1
  Add/1 -> Gain/1
  Product4/1 -> Gain3/1
  u1/1 -> Add2/1, Gain5/1
  Integrator13/1 -> x/1
  Product6/1 -> Add1/2
  Sin2/1 -> Product1/1
  Product8/1 -> Gain6/1
  Sin/1 -> Product/2
  Cos2/1 -> Product5/2
  Product3/1 -> Integrator22/1
  Subtract/1 -> Gain1/1
  Gain3/1 -> Add3/3

== system FBL_UAV_Final_All/Fixed-Gain PID/square wave1 ==
  Scope : Scope
  Step : Step  Time=4  SampleTime=0
  Step1 : Step  Time=8  After=-1  SampleTime=0
  Step2 : Step  Time=10  After=-1  SampleTime=0
  Sum6 : Sum  Inputs=|++++
  new : Step  Time=2  SampleTime=0.1
  Out1 : Outport
  wires:
  Sum6/1 -> Out1/1, Scope/1
  Step/1 -> Sum6/2
  new/1 -> Sum6/1
  Step1/1 -> Sum6/3
  Step2/1 -> Sum6/4

== system FBL_UAV_Final_All/LMPC/IAE Calculation1 ==
  In1 : Inport
  Abs : Abs  SaturateOnIntegerOverflow=off
  Integrator6 : Integrator
  Out1 : Outport
  wires:
  Abs/1 -> Integrator6/1
  Integrator6/1 -> Out1/1
  In1/1 -> Abs/1

== system FBL_UAV_Final_All/LMPC/ISE Calculation_z ==
  In1 : Inport
  Integrator6 : Integrator
  Square : Math  Operator=square
  ISE : Outport
  wires:
  Square/1 -> Integrator6/1
  Integrator6/1 -> ISE/1
  In1/1 -> Square/1

== system FBL_UAV_Final_All/LMPC/RMSE Calculation_altitude ==
  In1 : Inport
  Gain : Gain  Gain=1/3435
  Memory : Memory
  Sqrt : Sqrt
  Square : Math  Operator=square
  Sum : Sum  Inputs=|++
  Out1 : Outport
  wires:
  In1/1 -> Square/1
  Square/1 -> Sum/1
  Memory/1 -> Sum/2
  Sum/1 -> Gain/1
  Gain/1 -> Sqrt/1, Memory/1
  Sqrt/1 -> Out1/1

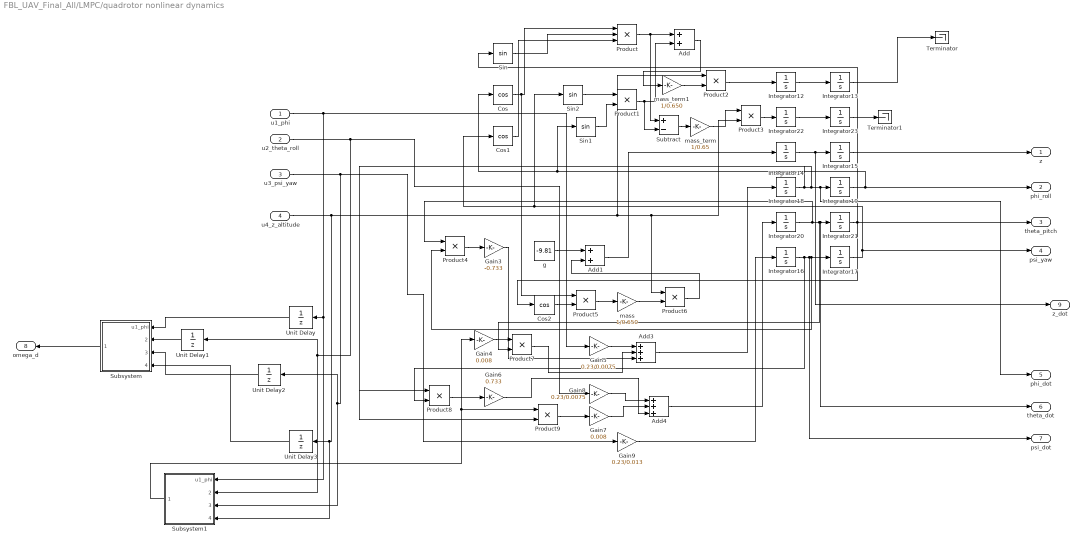
== system FBL_UAV_Final_All/LMPC/quadrotor nonlinear dynamics ==
  u1_phi : Inport
  u2_theta_roll : Inport  Port=2
  u3_psi_yaw : Inport  Port=3
  u4_z_altitude : Inport  Port=4
  Add : Sum
  Add1 : Sum
  Add3 : Sum  Inputs=+++
  Add4 : Sum  Inputs=+++
  Cos : Trigonometry  Operator=cos
  Cos1 : Trigonometry  Operator=cos
  Cos2 : Trigonometry  Operator=cos
  Gain3 : Gain  Gain=-0.733
  Gain4 : Gain  Gain=0.008
  Gain5 : Gain  Gain=0.23/0.0075
  Gain6 : Gain  Gain=0.733
  Gain7 : Gain  Gain=0.008
  Gain8 : Gain  Gain=0.23/0.0075
  Gain9 : Gain  Gain=0.23/0.013
  Integrator{12..15,18,20,22..23} (8 alike) : Integrator
  Integrator16 : Integrator  LowerSaturationLimit=0
  Integrator17 : Integrator  InitialCondition=1  LowerSaturationLimit=0
  Integrator19 : Integrator  InitialCondition=1  LowerSaturationLimit=0
  Integrator21 : Integrator  InitialCondition=1  LowerSaturationLimit=0
  Product : Product  Inputs=3
  Product{1..9} (9 alike) : Product
  Sin : Trigonometry
  Sin1 : Trigonometry
  Sin2 : Trigonometry
  Subsystem : Subsystem
  Subsystem1 : Subsystem
  Subtract : Sum  Inputs=+-
  Terminator : Terminator
  Terminator1 : Terminator
  Unit Delay{,1..3} (4 alike) : UnitDelay  SampleTime=-1  HasFrameUpgradeWarning=on
  g : Constant  Value=-9.81
  mass : Gain  Gain=1/0.650
  mass_term : Gain  Gain=1/0.65
  mass_term1 : Gain  Gain=1/0.650
  z : Outport
  phi_roll : Outport  Port=2
  theta_pitch : Outport  Port=3
  psi_yaw : Outport  Port=4
  phi_dot : Outport  Port=5
  theta_dot : Outport  Port=6
  psi_dot : Outport  Port=7
  omega_d : Outport  Port=8
  z_dot : Outport  Port=9
  wires:
  Gain9/1 -> Integrator16/1
  Product9/1 -> Gain7/1
  Gain6/1 -> Add4/3
  Add3/1 -> Integrator18/1
  Add4/1 -> Integrator20/1
  Gain7/1 -> Add4/2
  Gain4/1 -> Product7/1
  Product7/1 -> Add3/2
  Product1/1 -> Subtract/2, Add/2
  g/1 -> Add1/1
  mass_term/1 -> Product3/1
  Integrator18/1 -> Product9/2, Product8/1, phi_dot/1, Integrator19/1
  mass/1 -> Product6/2
  Gain8/1 -> Add4/1
  mass_term1/1 -> Product2/2
  Gain5/1 -> Add3/1
  Product5/1 -> mass/1
  Integrator12/1 -> Integrator13/1
  Product/1 -> Subtract/1, Add/1
  Product2/1 -> Integrator12/1
  Integrator15/1 -> z/1
  Integrator22/1 -> Integrator23/1
  Add1/1 -> Integrator14/1
  Integrator14/1 -> z_dot/1, Integrator15/1
  Cos1/1 -> Product/3
  Cos/1 -> Product5/1, Product/1
  Integrator17/1 -> Sin2/1, Cos1/1, psi_yaw/1
  Sin1/1 -> Product1/2
  Integrator20/1 -> theta_dot/1, Integrator21/1, Product7/2, Product4/1
  Integrator16/1 -> Product8/2, Product4/2, Integrator17/1, psi_dot/1
  Integrator21/1 -> theta_pitch/1, Cos2/1, Sin/1
  Add/1 -> mass_term1/1
  Product4/1 -> Gain3/1
  Product6/1 -> Add1/2
  Sin2/1 -> Product1/1
  Product8/1 -> Gain6/1
  Sin/1 -> Product/2
  Cos2/1 -> Product5/2
  Product3/1 -> Integrator22/1
  Subtract/1 -> mass_term/1
  Gain3/1 -> Add3/3
  Integrator19/1 -> Sin1/1, Cos/1, phi_roll/1
  u1_phi/1 -> Subsystem1/1(u1_phi), Unit Delay/1, Gain5/1
  u4_z_altitude/1 -> Product3/2, Product6/1, Product2/1, Subsystem1/4(u4_z_altitude), Unit Delay3/1
  u3_psi_yaw/1 -> Subsystem1/3(u3_psi_yaw), Unit Delay2/1, Gain9/1
  u2_theta_roll/1 -> Subsystem1/2(u2_theta_roll), Unit Delay1/1, Gain8/1
  Unit Delay/1 -> Subsystem/1(u1_phi)
  Unit Delay1/1 -> Subsystem/2(u2_theta_roll)
  Unit Delay2/1 -> Subsystem/3(u3_psi_yaw)
  Unit Delay3/1 -> Subsystem/4(u4_z_altitude)
  Integrator13/1 -> Terminator/1
  Integrator23/1 -> Terminator1/1
  Subsystem/1(omega_d) -> omega_d/1
  Subsystem1/1(omega_d) -> Product9/1, Gain4/1

== system FBL_UAV_Final_All/LMPC/square wave1 ==
  Scope : Scope
  Step : Step  Time=4  SampleTime=0
  Step1 : Step  Time=8  After=-1  SampleTime=0
  Step2 : Step  Time=10  After=-1  SampleTime=0
  Sum6 : Sum  Inputs=|++++
  new : Step  Time=2  SampleTime=0.1
  Out1 : Outport
  wires:
  Sum6/1 -> Out1/1, Scope/1
  Step/1 -> Sum6/2
  new/1 -> Sum6/1
  Step1/1 -> Sum6/3
  Step2/1 -> Sum6/4

== system FBL_UAV_Final_All/LQR/IAE Calculation1 ==
  In1 : Inport
  Abs : Abs  SaturateOnIntegerOverflow=off
  Integrator6 : Integrator
  Out1 : Outport
  wires:
  Abs/1 -> Integrator6/1
  Integrator6/1 -> Out1/1
  In1/1 -> Abs/1

== system FBL_UAV_Final_All/LQR/IAE Calculation2 ==
  In1 : Inport
  Abs : Abs  SaturateOnIntegerOverflow=off
  Integrator6 : Integrator
  Out1 : Outport
  wires:
  Abs/1 -> Integrator6/1
  Integrator6/1 -> Out1/1
  In1/1 -> Abs/1

== system FBL_UAV_Final_All/LQR/ISE Calculation_z ==
  In1 : Inport
  Integrator6 : Integrator
  Square : Math  Operator=square
  ISE : Outport
  wires:
  Square/1 -> Integrator6/1
  Integrator6/1 -> ISE/1
  In1/1 -> Square/1

== system FBL_UAV_Final_All/LQR/ISE Calculation_z1 ==
  In1 : Inport
  Integrator6 : Integrator
  Square : Math  Operator=square
  ISE : Outport
  wires:
  Square/1 -> Integrator6/1
  Integrator6/1 -> ISE/1
  In1/1 -> Square/1

== system FBL_UAV_Final_All/LQR/RMSE Calculation_altitude ==
  In1 : Inport
  Gain : Gain  Gain=1/3435
  Memory : Memory
  Sqrt : Sqrt
  Square : Math  Operator=square
  Sum : Sum  Inputs=|++
  Out1 : Outport
  wires:
  In1/1 -> Square/1
  Square/1 -> Sum/1
  Memory/1 -> Sum/2
  Sum/1 -> Gain/1
  Gain/1 -> Sqrt/1, Memory/1
  Sqrt/1 -> Out1/1

== system FBL_UAV_Final_All/LQR/RMSE Calculation_altitude1 ==
  In1 : Inport
  Gain : Gain  Gain=1/3435
  Memory : Memory
  Sqrt : Sqrt
  Square : Math  Operator=square
  Sum : Sum  Inputs=|++
  Out1 : Outport
  wires:
  In1/1 -> Square/1
  Square/1 -> Sum/1
  Memory/1 -> Sum/2
  Sum/1 -> Gain/1
  Gain/1 -> Sqrt/1, Memory/1
  Sqrt/1 -> Out1/1

== system FBL_UAV_Final_All/LQR/Subsystem5 ==
  In1 : Inport
  Gain : Gain  Gain=1/3435
  Memory : Memory
  Sqrt : Sqrt
  Square : Math  Operator=square
  Sum : Sum  Inputs=|++
  Out1 : Outport
  wires:
  In1/1 -> Square/1
  Square/1 -> Sum/1
  Memory/1 -> Sum/2
  Sum/1 -> Gain/1
  Gain/1 -> Sqrt/1, Memory/1
  Sqrt/1 -> Out1/1

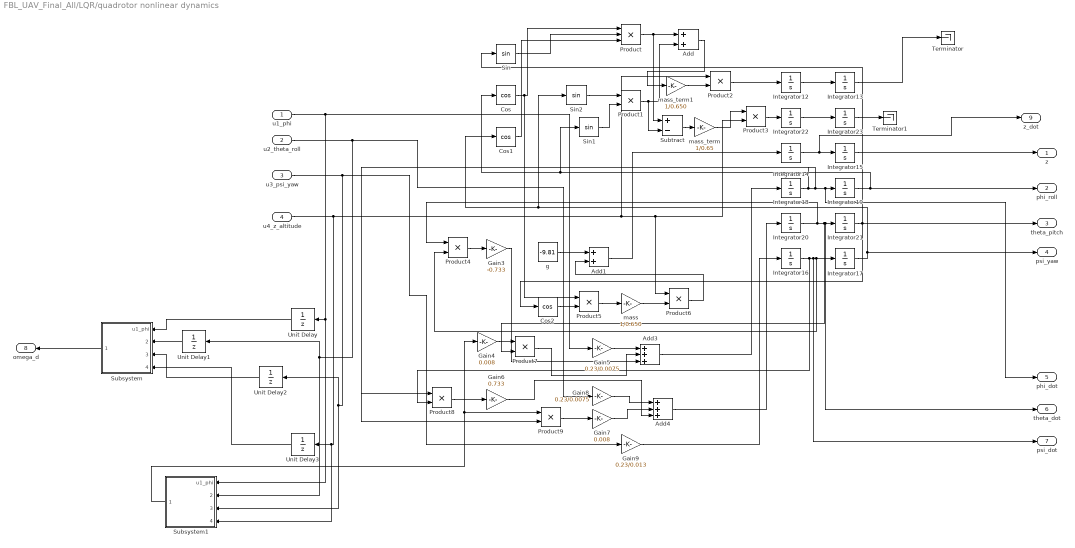
== system FBL_UAV_Final_All/LQR/quadrotor nonlinear dynamics ==
  u1_phi : Inport
  u2_theta_roll : Inport  Port=2
  u3_psi_yaw : Inport  Port=3
  u4_z_altitude : Inport  Port=4
  Add : Sum
  Add1 : Sum
  Add3 : Sum  Inputs=+++
  Add4 : Sum  Inputs=+++
  Cos : Trigonometry  Operator=cos
  Cos1 : Trigonometry  Operator=cos
  Cos2 : Trigonometry  Operator=cos
  Gain3 : Gain  Gain=-0.733
  Gain4 : Gain  Gain=0.008
  Gain5 : Gain  Gain=0.23/0.0075
  Gain6 : Gain  Gain=0.733
  Gain7 : Gain  Gain=0.008
  Gain8 : Gain  Gain=0.23/0.0075
  Gain9 : Gain  Gain=0.23/0.013
  Integrator{12..15,18,20,22..23} (8 alike) : Integrator
  Integrator16 : Integrator  LowerSaturationLimit=0
  Integrator17 : Integrator  InitialCondition=1  LowerSaturationLimit=0
  Integrator19 : Integrator  InitialCondition=1  LowerSaturationLimit=0
  Integrator21 : Integrator  InitialCondition=1  LowerSaturationLimit=0
  Product : Product  Inputs=3
  Product{1..9} (9 alike) : Product
  Sin : Trigonometry
  Sin1 : Trigonometry
  Sin2 : Trigonometry
  Subsystem : Subsystem
  Subsystem1 : Subsystem
  Subtract : Sum  Inputs=+-
  Terminator : Terminator
  Terminator1 : Terminator
  Unit Delay{,1..3} (4 alike) : UnitDelay  SampleTime=-1  HasFrameUpgradeWarning=on
  g : Constant  Value=-9.81
  mass : Gain  Gain=1/0.650
  mass_term : Gain  Gain=1/0.65
  mass_term1 : Gain  Gain=1/0.650
  z : Outport
  phi_roll : Outport  Port=2
  theta_pitch : Outport  Port=3
  psi_yaw : Outport  Port=4
  phi_dot : Outport  Port=5
  theta_dot : Outport  Port=6
  psi_dot : Outport  Port=7
  omega_d : Outport  Port=8
  z_dot : Outport  Port=9
  wires:
  Gain9/1 -> Integrator16/1
  Product9/1 -> Gain7/1
  Gain6/1 -> Add4/3
  Add3/1 -> Integrator18/1
  Add4/1 -> Integrator20/1
  Gain7/1 -> Add4/2
  Gain4/1 -> Product7/1
  Product7/1 -> Add3/2
  Product1/1 -> Subtract/2, Add/2
  g/1 -> Add1/1
  mass_term/1 -> Product3/1
  Integrator18/1 -> Product9/2, Product8/1, phi_dot/1, Integrator19/1
  mass/1 -> Product6/2
  Gain8/1 -> Add4/1
  mass_term1/1 -> Product2/2
  Gain5/1 -> Add3/1
  Product5/1 -> mass/1
  Integrator12/1 -> Integrator13/1
  Product/1 -> Subtract/1, Add/1
  Product2/1 -> Integrator12/1
  Integrator15/1 -> z/1
  Integrator22/1 -> Integrator23/1
  Add1/1 -> Integrator14/1
  Integrator14/1 -> z_dot/1, Integrator15/1
  Cos1/1 -> Product/3
  Cos/1 -> Product5/1, Product/1
  Integrator17/1 -> Sin2/1, Cos1/1, psi_yaw/1
  Sin1/1 -> Product1/2
  Integrator20/1 -> Integrator21/1, theta_dot/1, Product7/2, Product4/1
  Integrator16/1 -> Product8/2, Product4/2, Integrator17/1, psi_dot/1
  Integrator21/1 -> theta_pitch/1, Cos2/1, Sin/1
  Add/1 -> mass_term1/1
  Product4/1 -> Gain3/1
  Product6/1 -> Add1/2
  Sin2/1 -> Product1/1
  Product8/1 -> Gain6/1
  Sin/1 -> Product/2
  Cos2/1 -> Product5/2
  Product3/1 -> Integrator22/1
  Subtract/1 -> mass_term/1
  Gain3/1 -> Add3/3
  Integrator19/1 -> Sin1/1, Cos/1, phi_roll/1
  u1_phi/1 -> Subsystem1/1(u1_phi), Unit Delay/1, Gain5/1
  u4_z_altitude/1 -> Product3/2, Product6/1, Product2/1, Subsystem1/4(u4_z_altitude), Unit Delay3/1
  u3_psi_yaw/1 -> Subsystem1/3(u3_psi_yaw), Unit Delay2/1, Gain9/1
  u2_theta_roll/1 -> Subsystem1/2(u2_theta_roll), Unit Delay1/1, Gain8/1
  Unit Delay/1 -> Subsystem/1(u1_phi)
  Unit Delay1/1 -> Subsystem/2(u2_theta_roll)
  Unit Delay2/1 -> Subsystem/3(u3_psi_yaw)
  Unit Delay3/1 -> Subsystem/4(u4_z_altitude)
  Integrator13/1 -> Terminator/1
  Integrator23/1 -> Terminator1/1
  Subsystem/1(omega_d) -> omega_d/1
  Subsystem1/1(omega_d) -> Product9/1, Gain4/1

== system FBL_UAV_Final_All/LQR/square wave1 ==
  Scope : Scope
  Step : Step  Time=4  SampleTime=0
  Step1 : Step  Time=8  After=-1  SampleTime=0
  Step2 : Step  Time=10  After=-1  SampleTime=0
  Sum6 : Sum  Inputs=|++++
  new : Step  Time=2  SampleTime=0.1
  Out1 : Outport
  wires:
  Sum6/1 -> Out1/1, Scope/1
  Step/1 -> Sum6/2
  new/1 -> Sum6/1
  Step1/1 -> Sum6/3
  Step2/1 -> Sum6/4
